simulink model "shoot_and_inference_task"  (Simulink 3.00)
libraries: logiclib x16, langlib x8, genlib x1
settings Model: MaskType=REX sequence  MaskIconFrame=on  MaskIconOpaque=on  MaskIconRotate=none  MaskIconUnits=autoscale

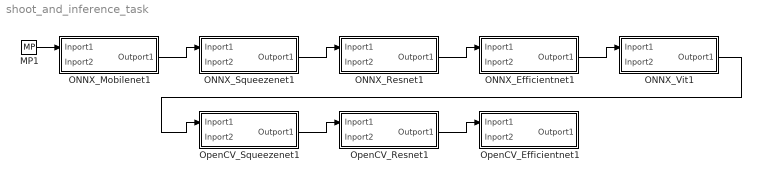
== system shoot_and_inference_task ==
  MP1 : genlib/MP  BSTATE=off  pwidth=1  RPTF=off
  ONNX_Efficientnet1 : Subsystem
      mask Type: REX sequence
  ONNX_Mobilenet1 : Subsystem
      mask Type: REX sequence
  ONNX_Resnet1 : Subsystem
      mask Type: REX sequence
  ONNX_Squeezenet1 : Subsystem
      mask Type: REX sequence
  ONNX_Vit1 : Subsystem
      mask Type: REX sequence
  OpenCV_Efficientnet1 : Subsystem
      mask Type: REX sequence
  OpenCV_Resnet1 : Subsystem
      mask Type: REX sequence
  OpenCV_Squeezenet1 : Subsystem
      mask Type: REX sequence
  wires:
  MP1/1 -> ONNX_Mobilenet1/1(Inport1)
  ONNX_Efficientnet1/1(Outport1) -> ONNX_Vit1/1(Inport1)
  ONNX_Mobilenet1/1(Outport1) -> ONNX_Squeezenet1/1(Inport1)
  ONNX_Resnet1/1(Outport1) -> ONNX_Efficientnet1/1(Inport1)
  ONNX_Squeezenet1/1(Outport1) -> ONNX_Resnet1/1(Inport1)
  ONNX_Vit1/1(Outport1) -> OpenCV_Squeezenet1/1(Inport1)
  OpenCV_Resnet1/1(Outport1) -> OpenCV_Efficientnet1/1(Inport1)
  OpenCV_Squeezenet1/1(Outport1) -> OpenCV_Resnet1/1(Inport1)

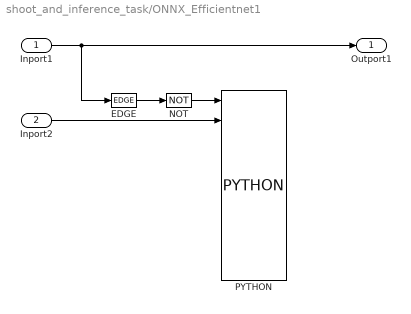
== system shoot_and_inference_task/ONNX_Efficientnet1 ==
  Inport1 : Inport  Port=1  OutDataTypeStr=Inherit: auto
  Inport2 : Inport  Port=2  OutDataTypeStr=Inherit: auto
  EDGE : logiclib/EDGE  iedge=1: Rising edge
  NOT : logiclib/NOT
  PYTHON : langlib/PYTHON  srcname=shoot_and_inference.py  embedded=on  p0=/mnt/external_hdd/ShootAndInferenceRexTest  p1=efficientnet_b0  p2=onnxruntime
  Outport1 : Outport  Port=1  OutDataTypeStr=Inherit: auto
  wires:
  EDGE/1 -> NOT/1
  Inport1/1 -> EDGE/1, Outport1/1
  Inport2/1 -> PYTHON/3
  NOT/1 -> PYTHON/1

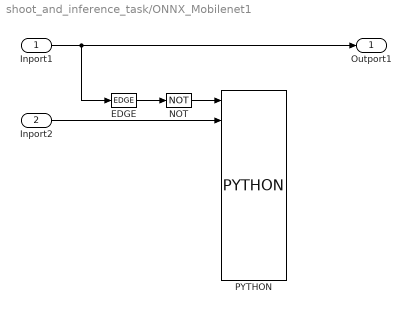
== system shoot_and_inference_task/ONNX_Mobilenet1 ==
  Inport1 : Inport  Port=1  OutDataTypeStr=Inherit: auto
  Inport2 : Inport  Port=2  OutDataTypeStr=Inherit: auto
  EDGE : logiclib/EDGE  iedge=1: Rising edge
  NOT : logiclib/NOT
  PYTHON : langlib/PYTHON  srcname=shoot_and_inference.py  embedded=on  p0=/mnt/external_hdd/ShootAndInferenceRexTest  p1=mobilenetv2  p2=onnxruntime
  Outport1 : Outport  Port=1  OutDataTypeStr=Inherit: auto
  wires:
  EDGE/1 -> NOT/1
  Inport1/1 -> EDGE/1, Outport1/1
  Inport2/1 -> PYTHON/3
  NOT/1 -> PYTHON/1

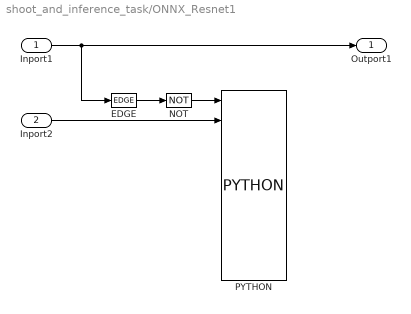
== system shoot_and_inference_task/ONNX_Resnet1 ==
  Inport1 : Inport  Port=1  OutDataTypeStr=Inherit: auto
  Inport2 : Inport  Port=2  OutDataTypeStr=Inherit: auto
  EDGE : logiclib/EDGE  iedge=1: Rising edge
  NOT : logiclib/NOT
  PYTHON : langlib/PYTHON  srcname=shoot_and_inference.py  embedded=on  p0=/mnt/external_hdd/ShootAndInferenceRexTest  p1=resnet50  p2=onnxruntime
  Outport1 : Outport  Port=1  OutDataTypeStr=Inherit: auto
  wires:
  EDGE/1 -> NOT/1
  Inport1/1 -> EDGE/1, Outport1/1
  Inport2/1 -> PYTHON/3
  NOT/1 -> PYTHON/1

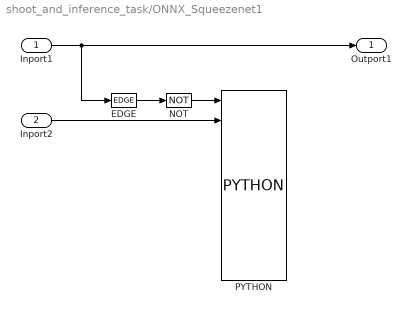
== system shoot_and_inference_task/ONNX_Squeezenet1 ==
  Inport1 : Inport  Port=1  OutDataTypeStr=Inherit: auto
  Inport2 : Inport  Port=2  OutDataTypeStr=Inherit: auto
  EDGE : logiclib/EDGE  iedge=1: Rising edge
  NOT : logiclib/NOT
  PYTHON : langlib/PYTHON  srcname=shoot_and_inference.py  embedded=on  p0=/mnt/external_hdd/ShootAndInferenceRexTest  p1=squeezenet  p2=onnxruntime
  Outport1 : Outport  Port=1  OutDataTypeStr=Inherit: auto
  wires:
  EDGE/1 -> NOT/1
  Inport1/1 -> EDGE/1, Outport1/1
  Inport2/1 -> PYTHON/3
  NOT/1 -> PYTHON/1

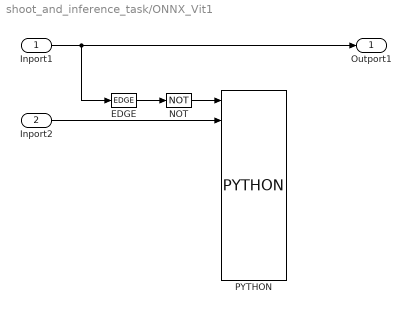
== system shoot_and_inference_task/ONNX_Vit1 ==
  Inport1 : Inport  Port=1  OutDataTypeStr=Inherit: auto
  Inport2 : Inport  Port=2  OutDataTypeStr=Inherit: auto
  EDGE : logiclib/EDGE  iedge=1: Rising edge
  NOT : logiclib/NOT
  PYTHON : langlib/PYTHON  srcname=shoot_and_inference.py  embedded=on  p0=/mnt/external_hdd/ShootAndInferenceRexTest  p1=vit_b16  p2=onnxruntime
  Outport1 : Outport  Port=1  OutDataTypeStr=Inherit: auto
  wires:
  EDGE/1 -> NOT/1
  Inport1/1 -> EDGE/1, Outport1/1
  Inport2/1 -> PYTHON/3
  NOT/1 -> PYTHON/1

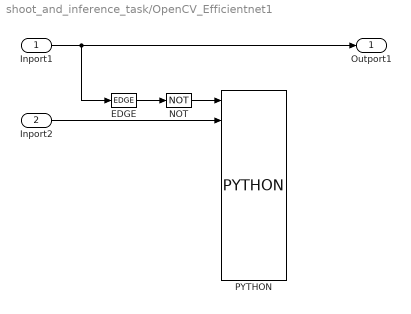
== system shoot_and_inference_task/OpenCV_Efficientnet1 ==
  Inport1 : Inport  Port=1  OutDataTypeStr=Inherit: auto
  Inport2 : Inport  Port=2  OutDataTypeStr=Inherit: auto
  EDGE : logiclib/EDGE  iedge=1: Rising edge
  NOT : logiclib/NOT
  PYTHON : langlib/PYTHON  srcname=shoot_and_inference.py  embedded=on  p0=/mnt/external_hdd/ShootAndInferenceRexTest  p1=efficientnet_b0  p2=opencv
  Outport1 : Outport  Port=1  OutDataTypeStr=Inherit: auto
  wires:
  EDGE/1 -> NOT/1
  Inport1/1 -> EDGE/1, Outport1/1
  Inport2/1 -> PYTHON/3
  NOT/1 -> PYTHON/1

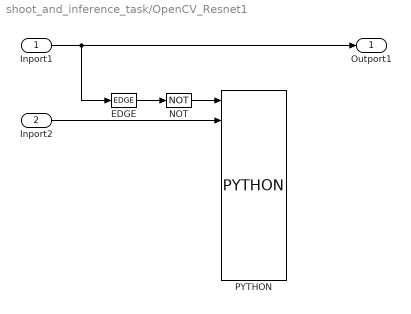
== system shoot_and_inference_task/OpenCV_Resnet1 ==
  Inport1 : Inport  Port=1  OutDataTypeStr=Inherit: auto
  Inport2 : Inport  Port=2  OutDataTypeStr=Inherit: auto
  EDGE : logiclib/EDGE  iedge=1: Rising edge
  NOT : logiclib/NOT
  PYTHON : langlib/PYTHON  srcname=shoot_and_inference.py  embedded=on  p0=/mnt/external_hdd/ShootAndInferenceRexTest  p1=resnet50  p2=opencv
  Outport1 : Outport  Port=1  OutDataTypeStr=Inherit: auto
  wires:
  EDGE/1 -> NOT/1
  Inport1/1 -> EDGE/1, Outport1/1
  Inport2/1 -> PYTHON/3
  NOT/1 -> PYTHON/1

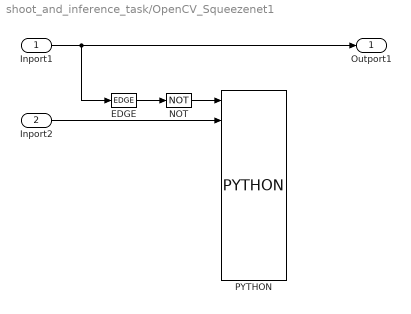
== system shoot_and_inference_task/OpenCV_Squeezenet1 ==
  Inport1 : Inport  Port=1  OutDataTypeStr=Inherit: auto
  Inport2 : Inport  Port=2  OutDataTypeStr=Inherit: auto
  EDGE : logiclib/EDGE  iedge=1: Rising edge
  NOT : logiclib/NOT
  PYTHON : langlib/PYTHON  srcname=shoot_and_inference.py  embedded=on  p0=/mnt/external_hdd/ShootAndInferenceRexTest  p1=squeezenet  p2=opencv
  Outport1 : Outport  Port=1  OutDataTypeStr=Inherit: auto
  wires:
  EDGE/1 -> NOT/1
  Inport1/1 -> EDGE/1, Outport1/1
  Inport2/1 -> PYTHON/3
  NOT/1 -> PYTHON/1
